simulink model "EPS_Exp_07"  (R2014a)
settings: Solver=ode45  StartTime=0.0  StopTime=0.05  RelTol=1e-3
undefined symbols (not defined in the file): D1, Delta
libraries: powerlib x11
settings Model: Creator=dell  LastModifiedBy=dell

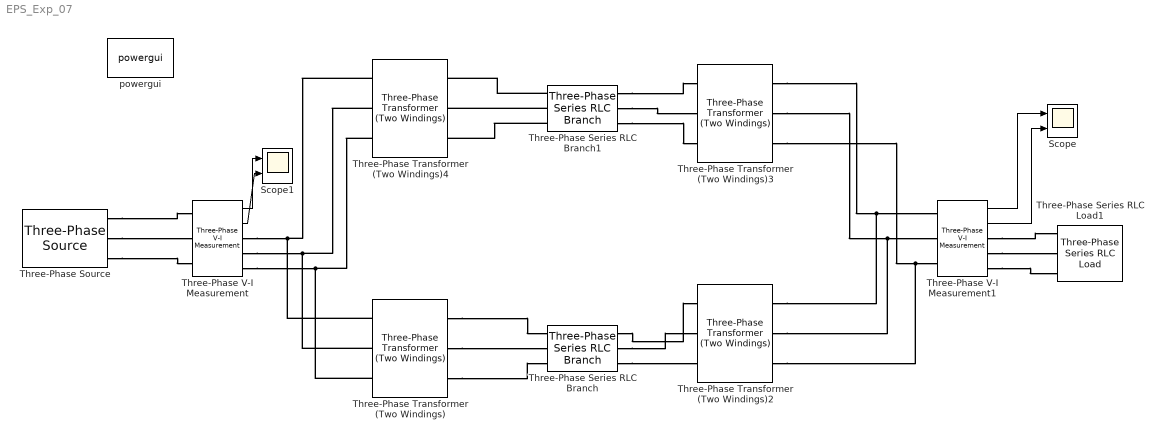
== system EPS_Exp_07 ==
  Scope : Scope  NumInputPorts=2
      settings: YMin=-5500~-0.9  YMax=5500~0.9  SampleInput=on  SampleTime=1e-6
  Scope1 : Scope  NumInputPorts=2
      settings: YMin=-15000~-5  YMax=15000~5  SampleInput=on  SampleTime=1e-6
  Three-Phase Series RLC Branch : powerlib/Elements/Three-Phase Series RLC Branch  LConnTagsString=A|B|C  RConnTagsString=A|B|C  BranchType=RLC  Resistance=1e-3  Inductance=65.43/(2*pi*50)  Capacitance=0  Measurements=None
  Three-Phase Series RLC Branch1 : powerlib/Elements/Three-Phase Series RLC Branch  LConnTagsString=A|B|C  RConnTagsString=A|B|C  BranchType=RLC  Resistance=1e-3  Inductance=48.4/(2*pi*50)  Capacitance=0  Measurements=None
  Three-Phase Series RLC Load1 : powerlib/Elements/Three-Phase Series RLC Load  LConnTagsString=A|B|C  Configuration=Y (grounded)  NominalVoltage=10.45e3  NominalFrequency=50  ActivePower=34.2e6  InductivePower=45.6e6  CapacitivePower=0  Measurements=None  LoadType=constant Z
  Three-Phase Transformer (Two Windings) : powerlib/Elements/Three-Phase Transformer (Two Windings)  Winding1Connection=Delta (D1)  UNITS=pu  NominalPower=[ 40e6 , 50 ]  Winding1=[ 22e3 , 0.002 , 0.064 ]  Winding2Connection=Delta (D1)  Winding2=[ 110e3 , 0.002 , 0.064 ]  SetSaturation=off  Rm=500  Lm=500  Saturation=[ 0,0 ; 0.0024,1.2 ; 1.0,1.52 ]  Hysteresis=off  DataFile='hysteresis'  SetInitialFlux=off  InitialFluxes=[ 0.8 , -0.8 , 0.7 ]  Measurements=None  MoreParameters=off  BreakLoop=off  DataType=off  TransfoNumber=1
  Three-Phase Transformer (Two Windings)2 : powerlib/Elements/Three-Phase Transformer (Two Windings)  Winding1Connection=Delta (D1)  UNITS=pu  NominalPower=[ 40e6 , 50 ]  Winding1=[ 110e3 , 0.002 , 0.08 ]  Winding2Connection=Yg  Winding2=[ 11e3 , 0.002 , 0.08 ]  SetSaturation=off  Rm=500  Lm=500  Saturation=[ 0,0 ; 0.0024,1.2 ; 1.0,1.52 ]  Hysteresis=off  DataFile='hysteresis'  SetInitialFlux=off  InitialFluxes=[ 0.8 , -0.8 , 0.7 ]  Measurements=None  MoreParameters=off  BreakLoop=off  DataType=off  TransfoNumber=1
  Three-Phase Transformer (Two Windings)3 : powerlib/Elements/Three-Phase Transformer (Two Windings)  Winding1Connection=Delta (D1)  UNITS=pu  NominalPower=[ 40e6 , 50 ]  Winding1=[ 220e3 , 0.002 , 0.06 ]  Winding2Connection=Yg  Winding2=[ 11e3 , 0.002 , 0.06 ]  SetSaturation=off  Rm=500  Lm=500  Saturation=[ 0,0 ; 0.0024,1.2 ; 1.0,1.52 ]  Hysteresis=off  DataFile='hysteresis'  SetInitialFlux=off  InitialFluxes=[ 0.8 , -0.8 , 0.7 ]  Measurements=None  MoreParameters=off  BreakLoop=off  DataType=off  TransfoNumber=1
  Three-Phase Transformer (Two Windings)4 : powerlib/Elements/Three-Phase Transformer (Two Windings)  Winding1Connection=Delta (D1)  UNITS=pu  NominalPower=[ 50e6 , 50 ]  Winding1=[ 22e3 , 0.002 , 0.1]  Winding2Connection=Delta (D1)  Winding2=[ 220e3 , 0.002 , 0.1 ]  SetSaturation=off  Rm=500  Lm=500  Saturation=[ 0,0 ; 0.0024,1.2 ; 1.0,1.52 ]  Hysteresis=off  DataFile='hysteresis'  SetInitialFlux=off  InitialFluxes=[ 0.8 , -0.8 , 0.7 ]  Measurements=None  MoreParameters=off  BreakLoop=off  DataType=off  TransfoNumber=1
  Three-Phase V-I Measurement : powerlib/Measurements/Three-Phase V-I Measurement  VoltageMeasurement=phase-to-ground  SetLabelV=off  LabelV=Vabc  Vpu=off  VpuLL=off  CurrentMeasurement=yes  SetLabelI=off  LabelI=Iabc  Ipu=on  Pbase=90e6  Vbase=22e3  OutputType=Complex  PhasorSimulation=off  PSBequivalent=0
  Three-Phase V-I Measurement1 : powerlib/Measurements/Three-Phase V-I Measurement  VoltageMeasurement=phase-to-ground  SetLabelV=off  LabelV=Vabc  Vpu=off  VpuLL=off  CurrentMeasurement=yes  SetLabelI=off  LabelI=Iabc  Ipu=on  Pbase=90e6  Vbase=22e3  OutputType=Complex  PhasorSimulation=off  PSBequivalent=0
  Three-Phase Source : powerlib/Electrical Sources/Three-Phase Source  Voltage=25e3  PhaseAngle=0  Frequency=50  InternalConnection=Yg  SpecifyImpedance=on  Resistance=0.8929  Inductance=16.58e-3  ShortCircuitLevel=90e6  BaseVoltage=22e3  XRratio=7  BusType=swing  Pref=0  Qref=0  Qmin=-inf  Qmax=inf
  powergui : powerlib/powergui  Priority=1  SimulationMode=Continuous  SolverType=Tustin  SampleTime=50e-6  frequency=60  SPID=off  DisableSnubberDevices=off  DisableRonSwitches=off  DisableVfSwitches=off  SwTol=0  Interpol=off  DisplayEquations=off  Ts=0  methode=off  frequencyindice=50  Pbase=100e6  ErrMax=1e-4  Iterations=50  UnitsV=kV  UnitsW=MW  FunctionMessages=off  echomessages=off  HookPort=off  EnableUseOfTLC=off  x0status=blocks  RestoreLinks=warning  ResistiveCurrentMeasurement=off  Frange=[0:2:500]  Ylog=off  Xlog=on  ShowGrid=off  save=off  variable=ZData  structure=0  ZoomFFT=off  StartTime=0.0  cycles=1  DisplayStyle=1  fundamental=60  FreqAxis=off  MaxFrequency=1000  frequencyindicesteady=1  RmsSteady=1  display=off
  wires:
  Three-Phase V-I Measurement/1 -> Scope1/1
  Three-Phase V-I Measurement1/1 -> Scope/1
  Three-Phase V-I Measurement1/2 -> Scope/2
  Three-Phase V-I Measurement/2 -> Scope1/2
  connections:
  Three-Phase Source/RConn1 -- Three-Phase V-I Measurement/LConn1
  Three-Phase Source/RConn2 -- Three-Phase V-I Measurement/LConn2
  Three-Phase Source/RConn3 -- Three-Phase V-I Measurement/LConn3
  Three-Phase V-I Measurement/RConn1 -- Three-Phase Transformer (Two Windings)4/LConn1 -- Three-Phase Transformer (Two Windings)/LConn1
  Three-Phase V-I Measurement/RConn2 -- Three-Phase Transformer (Two Windings)4/LConn2 -- Three-Phase Transformer (Two Windings)/LConn2
  Three-Phase V-I Measurement/RConn3 -- Three-Phase Transformer (Two Windings)4/LConn3 -- Three-Phase Transformer (Two Windings)/LConn3
  Three-Phase Series RLC Branch1/LConn1 -- Three-Phase Transformer (Two Windings)4/RConn1
  Three-Phase Series RLC Branch1/LConn2 -- Three-Phase Transformer (Two Windings)4/RConn2
  Three-Phase Series RLC Branch1/LConn3 -- Three-Phase Transformer (Two Windings)4/RConn3
  Three-Phase Series RLC Branch1/RConn1 -- Three-Phase Transformer (Two Windings)3/LConn1
  Three-Phase Series RLC Branch1/RConn2 -- Three-Phase Transformer (Two Windings)3/LConn2
  Three-Phase Series RLC Branch1/RConn3 -- Three-Phase Transformer (Two Windings)3/LConn3
  Three-Phase Series RLC Branch/RConn1 -- Three-Phase Transformer (Two Windings)2/LConn1
  Three-Phase Series RLC Branch/RConn2 -- Three-Phase Transformer (Two Windings)2/LConn2
  Three-Phase Series RLC Branch/RConn3 -- Three-Phase Transformer (Two Windings)2/LConn3
  Three-Phase Transformer (Two Windings)/RConn1 -- Three-Phase Series RLC Branch/LConn1
  Three-Phase Transformer (Two Windings)/RConn2 -- Three-Phase Series RLC Branch/LConn2
  Three-Phase Transformer (Two Windings)/RConn3 -- Three-Phase Series RLC Branch/LConn3
  Three-Phase Transformer (Two Windings)3/RConn1 -- Three-Phase Transformer (Two Windings)2/RConn1 -- Three-Phase V-I Measurement1/LConn1
  Three-Phase Transformer (Two Windings)3/RConn2 -- Three-Phase Transformer (Two Windings)2/RConn2 -- Three-Phase V-I Measurement1/LConn2
  Three-Phase Transformer (Two Windings)3/RConn3 -- Three-Phase Transformer (Two Windings)2/RConn3 -- Three-Phase V-I Measurement1/LConn3
  Three-Phase V-I Measurement1/RConn1 -- Three-Phase Series RLC Load1/LConn1
  Three-Phase V-I Measurement1/RConn2 -- Three-Phase Series RLC Load1/LConn2
  Three-Phase V-I Measurement1/RConn3 -- Three-Phase Series RLC Load1/LConn3
